simulink library "uavsimBlockset_VectorNorm"  (Simulink 8.4)
settings: Solver=ode45  StartTime=0.0  StopTime=10.0  RelTol=1e-3
settings Model: Creator=mstolle  LastModifiedBy=j.bolting

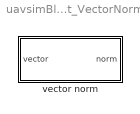
== system uavsimBlockset_VectorNorm ==
  vector norm : Subsystem

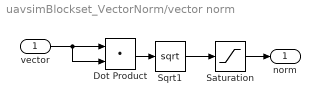
== system uavsimBlockset_VectorNorm/vector norm ==
  vector : Inport  OutDataTypeStr=double
  Dot Product : DotProduct  InputSameDT=on  OutDataTypeStr=Inherit: Inherit via internal rule
  Saturation : Saturate  UpperLimit=inf  LowerLimit=eps
  Sqrt1 : Sqrt  OutputSignalType=real  SaturateOnIntegerOverflow=on
  norm : Outport  OutDataTypeStr=double  PortDimensions=1
  wires:
  vector/1 -> Dot Product/2, Dot Product/1
  Dot Product/1 -> Sqrt1/1
  Sqrt1/1 -> Saturation/1
  Saturation/1 -> norm/1
